simulink model "Punto1d_real_velocidad_01Ktac"  (Simulink 7.5)
settings: Solver=ode45  StartTime=0  StopTime=10  MaxStep=0.01  RelTol=1e-3
settings Model: Creator=Nahuek  LastModifiedBy=Nahuek

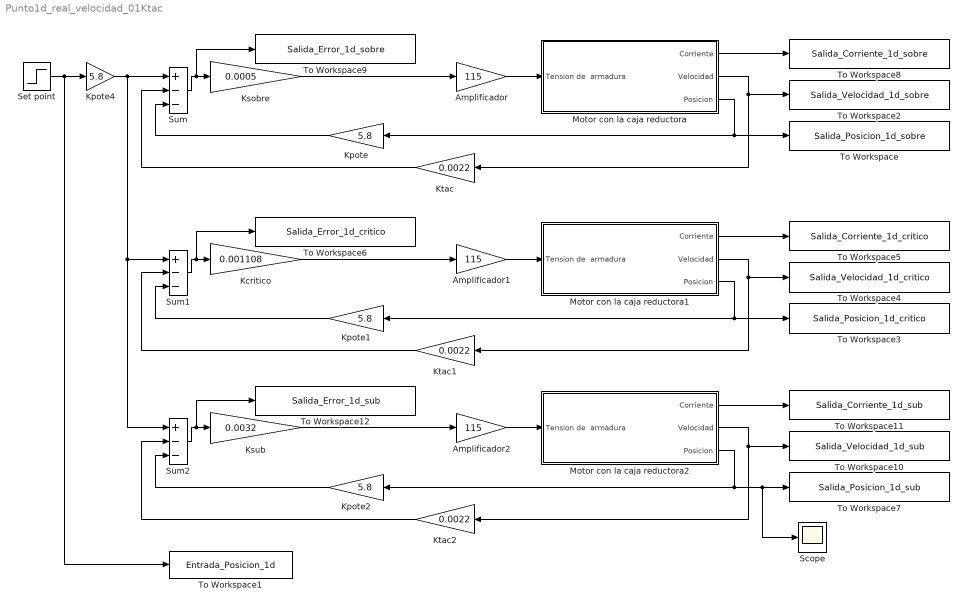
== system Punto1d_real_velocidad_01Ktac ==
  Amplificador : Gain  Gain=115  ParameterDataType=fixdt(1, 16)  ParameterScaling=2^0  OutDataType=fixdt(1, 16)  OutScaling=2^0
  Amplificador1 : Gain  Gain=115  ParameterDataType=fixdt(1, 16)  ParameterScaling=2^0  OutDataType=fixdt(1, 16)  OutScaling=2^0
  Amplificador2 : Gain  Gain=115  ParameterDataType=fixdt(1, 16)  ParameterScaling=2^0  OutDataType=fixdt(1, 16)  OutScaling=2^0
  Kcritico : Gain  Gain=0.001108  ParameterDataType=fixdt(1, 16)  ParameterScaling=2^0  OutDataType=fixdt(1, 16)  OutScaling=2^0
  Kpote{,1..2,4} (4 alike) : Gain  Gain=5.8  ParameterDataType=fixdt(1, 16)  ParameterScaling=2^0  OutDataType=fixdt(1, 16)  OutScaling=2^0
  Ksobre : Gain  Gain=0.0005  ParameterDataType=fixdt(1, 16)  ParameterScaling=2^0  OutDataType=fixdt(1, 16)  OutScaling=2^0
  Ksub : Gain  Gain=0.0032  ParameterDataType=fixdt(1, 16)  ParameterScaling=2^0  OutDataType=fixdt(1, 16)  OutScaling=2^0
  Ktac : Gain  Gain=0.0022  ParameterDataType=fixdt(1, 16)  ParameterScaling=2^0  OutDataType=fixdt(1, 16)  OutScaling=2^0
  Ktac1 : Gain  Gain=0.0022  ParameterDataType=fixdt(1, 16)  ParameterScaling=2^0  OutDataType=fixdt(1, 16)  OutScaling=2^0
  Ktac2 : Gain  Gain=0.0022  ParameterDataType=fixdt(1, 16)  ParameterScaling=2^0  OutDataType=fixdt(1, 16)  OutScaling=2^0
  Motor con la caja reductora : Subsystem
  Motor con la caja reductora1 : Subsystem
  Motor con la caja reductora2 : Subsystem
  Scope : Scope
  Set point : Step  Time=0  SampleTime=0
  Sum : Sum  Inputs=+--  OutDataType=fixdt(1, 16)  OutScaling=2^0
  Sum1 : Sum  Inputs=+--  OutDataType=fixdt(1, 16)  OutScaling=2^0
  Sum2 : Sum  Inputs=+--  OutDataType=fixdt(1, 16)  OutScaling=2^0
  To Workspace : ToWorkspace  VariableName=Salida_Posicion_1d_sobre  SampleTime=-1  SaveFormat=Structure With Time
  To Workspace1 : ToWorkspace  VariableName=Entrada_Posicion_1d  SampleTime=-1  SaveFormat=Structure With Time
  To Workspace10 : ToWorkspace  VariableName=Salida_Velocidad_1d_sub  SampleTime=-1  SaveFormat=Structure With Time
  To Workspace11 : ToWorkspace  VariableName=Salida_Corriente_1d_sub  SampleTime=-1  SaveFormat=Structure With Time
  To Workspace12 : ToWorkspace  VariableName=Salida_Error_1d_sub  SampleTime=-1  SaveFormat=Structure With Time
  To Workspace2 : ToWorkspace  VariableName=Salida_Velocidad_1d_sobre  SampleTime=-1  SaveFormat=Structure With Time
  To Workspace3 : ToWorkspace  VariableName=Salida_Posicion_1d_critico  SampleTime=-1  SaveFormat=Structure With Time
  To Workspace4 : ToWorkspace  VariableName=Salida_Velocidad_1d_critico  SampleTime=-1  SaveFormat=Structure With Time
  To Workspace5 : ToWorkspace  VariableName=Salida_Corriente_1d_critico  SampleTime=-1  SaveFormat=Structure With Time
  To Workspace6 : ToWorkspace  VariableName=Salida_Error_1d_critico  SampleTime=-1  SaveFormat=Structure With Time
  To Workspace7 : ToWorkspace  VariableName=Salida_Posicion_1d_sub  SampleTime=-1  SaveFormat=Structure With Time
  To Workspace8 : ToWorkspace  VariableName=Salida_Corriente_1d_sobre  SampleTime=-1  SaveFormat=Structure With Time
  To Workspace9 : ToWorkspace  VariableName=Salida_Error_1d_sobre  SampleTime=-1  SaveFormat=Structure With Time
  wires:
  Sum/1 -> Ksobre/1, To Workspace9/1
  Amplificador/1 -> Motor con la caja reductora/1(Tension de  armadura)
  Set point/1 -> Kpote4/1, To Workspace1/1
  Kpote4/1 -> Sum/1, Sum1/1, Sum2/1
  Kpote/1 -> Sum/3
  Motor con la caja reductora/1(Corriente) -> To Workspace8/1
  Ksobre/1 -> Amplificador/1
  Ktac/1 -> Sum/2
  Motor con la caja reductora/3(Posicion) -> Kpote/1, To Workspace/1
  Motor con la caja reductora/2(Velocidad) -> To Workspace2/1, Ktac/1
  Sum1/1 -> Kcritico/1, To Workspace6/1
  Amplificador1/1 -> Motor con la caja reductora1/1(Tension de  armadura)
  Kpote1/1 -> Sum1/3
  Motor con la caja reductora1/1(Corriente) -> To Workspace5/1
  Kcritico/1 -> Amplificador1/1
  Ktac1/1 -> Sum1/2
  Motor con la caja reductora1/3(Posicion) -> Kpote1/1, To Workspace3/1
  Motor con la caja reductora1/2(Velocidad) -> To Workspace4/1, Ktac1/1
  Sum2/1 -> Ksub/1, To Workspace12/1
  Amplificador2/1 -> Motor con la caja reductora2/1(Tension de  armadura)
  Kpote2/1 -> Sum2/3
  Motor con la caja reductora2/1(Corriente) -> To Workspace11/1
  Ksub/1 -> Amplificador2/1
  Ktac2/1 -> Sum2/2
  Motor con la caja reductora2/3(Posicion) -> Kpote2/1, To Workspace7/1, Scope/1
  Motor con la caja reductora2/2(Velocidad) -> To Workspace10/1, Ktac2/1

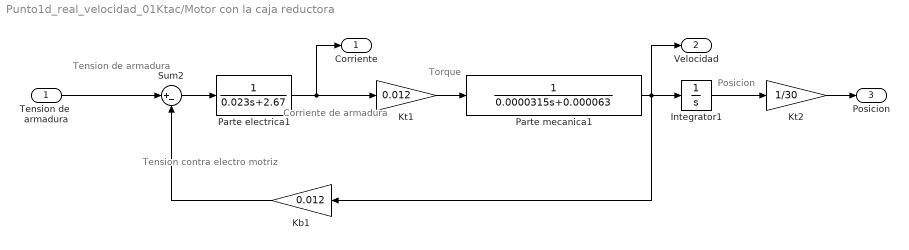
== system Punto1d_real_velocidad_01Ktac/Motor con la caja reductora ==
  note: Tension contra
      |  electro motriz
  note: Corriente de
      | armadura
  note: Torque
  note: Posicion
  note: Tension de
      |  armadura
  Tension de  armadura : Inport
  Integrator1 : Integrator
  Kb1 : Gain  Gain=0.012  ParameterDataType=fixdt(1, 16)  ParameterScaling=2^0  OutDataType=fixdt(1, 16)  OutScaling=2^0
  Kt1 : Gain  Gain=0.012  ParameterDataType=fixdt(1, 16)  ParameterScaling=2^0  OutDataType=fixdt(1, 16)  OutScaling=2^0
  Kt2 : Gain  Gain=1/30  ParameterDataType=fixdt(1, 16)  ParameterScaling=2^0  OutDataType=fixdt(1, 16)  OutScaling=2^0
  Parte electrica1 : TransferFcn  Denominator=[0.023 2.67]
  Parte mecanica1 : TransferFcn  Denominator=[0.0000315 0.000063]
  Sum2 : Sum  Inputs=|+-  OutDataType=fixdt(1, 16)  OutScaling=2^0
  Corriente : Outport
  Velocidad : Outport  Port=2
  Posicion : Outport  Port=3
  wires:
  Sum2/1 -> Parte electrica1/1
  Kt1/1 -> Parte mecanica1/1
  Parte electrica1/1 -> Kt1/1, Corriente/1
  Kb1/1 -> Sum2/2
  Parte mecanica1/1 -> Integrator1/1, Kb1/1, Velocidad/1
  Tension de  armadura/1 -> Sum2/1
  Kt2/1 -> Posicion/1
  Integrator1/1 -> Kt2/1

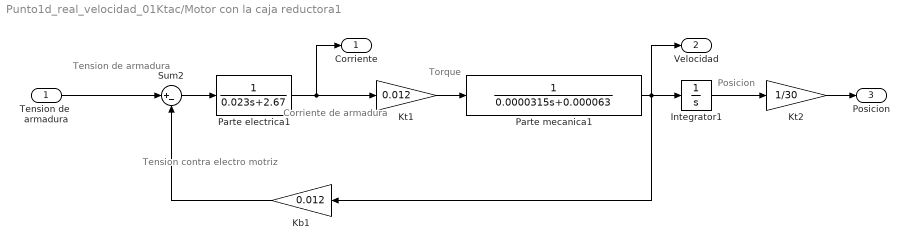
== system Punto1d_real_velocidad_01Ktac/Motor con la caja reductora1 ==
  note: Tension contra
      |  electro motriz
  note: Corriente de
      | armadura
  note: Torque
  note: Posicion
  note: Tension de
      |  armadura
  Tension de  armadura : Inport
  Integrator1 : Integrator
  Kb1 : Gain  Gain=0.012  ParameterDataType=fixdt(1, 16)  ParameterScaling=2^0  OutDataType=fixdt(1, 16)  OutScaling=2^0
  Kt1 : Gain  Gain=0.012  ParameterDataType=fixdt(1, 16)  ParameterScaling=2^0  OutDataType=fixdt(1, 16)  OutScaling=2^0
  Kt2 : Gain  Gain=1/30  ParameterDataType=fixdt(1, 16)  ParameterScaling=2^0  OutDataType=fixdt(1, 16)  OutScaling=2^0
  Parte electrica1 : TransferFcn  Denominator=[0.023 2.67]
  Parte mecanica1 : TransferFcn  Denominator=[0.0000315 0.000063]
  Sum2 : Sum  Inputs=|+-  OutDataType=fixdt(1, 16)  OutScaling=2^0
  Corriente : Outport
  Velocidad : Outport  Port=2
  Posicion : Outport  Port=3
  wires:
  Sum2/1 -> Parte electrica1/1
  Kt1/1 -> Parte mecanica1/1
  Parte electrica1/1 -> Kt1/1, Corriente/1
  Kb1/1 -> Sum2/2
  Parte mecanica1/1 -> Integrator1/1, Kb1/1, Velocidad/1
  Tension de  armadura/1 -> Sum2/1
  Kt2/1 -> Posicion/1
  Integrator1/1 -> Kt2/1

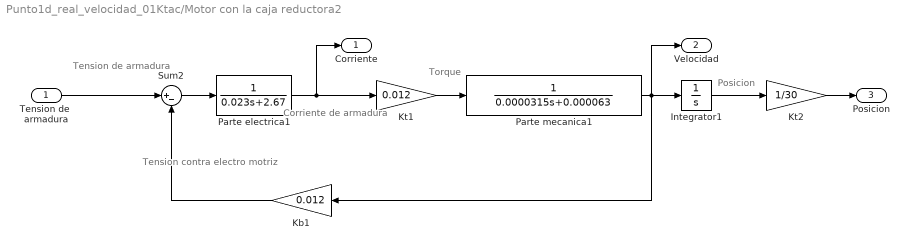
== system Punto1d_real_velocidad_01Ktac/Motor con la caja reductora2 ==
  note: Tension contra
      |  electro motriz
  note: Corriente de
      | armadura
  note: Torque
  note: Posicion
  note: Tension de
      |  armadura
  Tension de  armadura : Inport
  Integrator1 : Integrator
  Kb1 : Gain  Gain=0.012  ParameterDataType=fixdt(1, 16)  ParameterScaling=2^0  OutDataType=fixdt(1, 16)  OutScaling=2^0
  Kt1 : Gain  Gain=0.012  ParameterDataType=fixdt(1, 16)  ParameterScaling=2^0  OutDataType=fixdt(1, 16)  OutScaling=2^0
  Kt2 : Gain  Gain=1/30  ParameterDataType=fixdt(1, 16)  ParameterScaling=2^0  OutDataType=fixdt(1, 16)  OutScaling=2^0
  Parte electrica1 : TransferFcn  Denominator=[0.023 2.67]
  Parte mecanica1 : TransferFcn  Denominator=[0.0000315 0.000063]
  Sum2 : Sum  Inputs=|+-  OutDataType=fixdt(1, 16)  OutScaling=2^0
  Corriente : Outport
  Velocidad : Outport  Port=2
  Posicion : Outport  Port=3
  wires:
  Sum2/1 -> Parte electrica1/1
  Kt1/1 -> Parte mecanica1/1
  Parte electrica1/1 -> Kt1/1, Corriente/1
  Kb1/1 -> Sum2/2
  Parte mecanica1/1 -> Integrator1/1, Kb1/1, Velocidad/1
  Tension de  armadura/1 -> Sum2/1
  Kt2/1 -> Posicion/1
  Integrator1/1 -> Kt2/1
